simulink model "Second_order_simulink"  (R2020b)
settings: Solver=VariableStepAuto  StartTime=0.0  StopTime=100  RelTol=1e-3
settings Model: Creator=99003785  LastModifiedBy=99003785

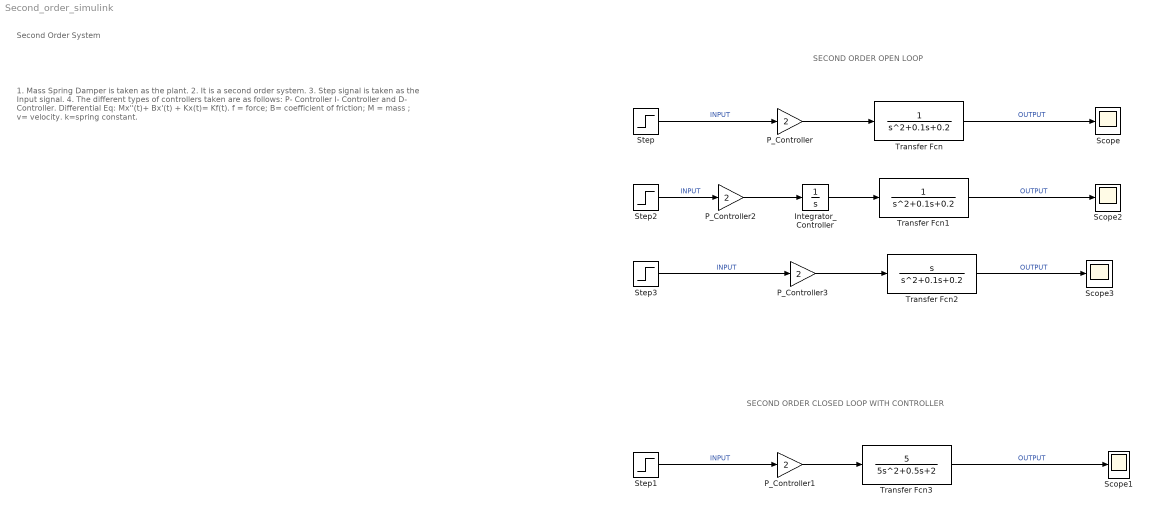
== system Second_order_simulink ==
  note: SECOND ORDER OPEN LOOP
  note: SECOND ORDER CLOSED LOOP WITH CONTROLLER
  note: 1. Mass Spring Damper is taken as the plant.
      | 2. It is a second order system.
      | 3. Step signal is taken as the Input signal.
      | 4. The different types of controllers taken are as follows:
      | P- Controller I- Controller and D- Controller.
      |
      | Differential Eq: Mx''(t)+ Bx'(t) + Kx(t)= Kf(t).
      | f = force; B= coefficient of friction; M = mass ;
      | v= velocity. k=spring constant.
  note: Second Order System
  Integrator_Controller : Integrator
  P_Controller{,1..3} (4 alike) : Gain  Gain=2
  Scope{,1..3} (4 alike) : Scope
  Step{,1..3} (4 alike) : Step  SampleTime=0
  Transfer Fcn : TransferFcn  Denominator=[1 0.1 0.2]
  Transfer Fcn1 : TransferFcn  Denominator=[1 0.1 0.2]
  Transfer Fcn2 : TransferFcn  Numerator=[1 0]  Denominator=[1 0.1 0.2]
  Transfer Fcn3 : TransferFcn  Numerator=[5]  Denominator=[5 0.5 2]
  wires:
  Step2/1 -> P_Controller2/1  "INPUT"
  P_Controller2/1 -> Integrator_Controller/1
  Step3/1 -> P_Controller3/1  "INPUT"
  Step1/1 -> P_Controller1/1  "INPUT"
  Transfer Fcn/1 -> Scope/1  "OUTPUT"
  Step/1 -> P_Controller/1  "INPUT"
  P_Controller/1 -> Transfer Fcn/1
  Transfer Fcn1/1 -> Scope2/1  "OUTPUT"
  Integrator_Controller/1 -> Transfer Fcn1/1
  P_Controller3/1 -> Transfer Fcn2/1
  Transfer Fcn2/1 -> Scope3/1  "OUTPUT"
  Transfer Fcn3/1 -> Scope1/1  "OUTPUT"
  P_Controller1/1 -> Transfer Fcn3/1
